simulink model "Electrical_System_2018b_obfs"  (R2019b)
settings: Solver=VariableStepAuto  StartTime=0.0  StopTime=5  RelTol=1e-3  AbsTol=1e-3  EnableMultiTasking=on
InitFcn:
  | Steady_State_Initialisation;
StopFcn:
  | %sscexplore(simlog);
  | %Logging
undefined symbols (not defined in the file): abrlhklxvp, aexgmhuedq, afmfmjnutg, afpphrjpnc, ahuxbyvruc, alarvljztt, amxnyqmnuw, aodrlwvqie, aolhmuplyq, aqpmguuqkg, auesgwirzl, aurophlnng, awamelrhru, ayfhvxflxn, azxkacuhqc, babszerikg, bawhdqanwq, bevoqecvei, bltjvqbchx, bmqsuewujl, bsmyqjfgnf, btvjbsmnve, bywgxqeadw, bziaduxaer, bzmcmdqocb, bzsvyvetat, ccsjnrbsih, cdvenygxwh, cedkrnslhx, cjheorclzs, cjrdshrtqx, ckhavyhcza, ckxewznhlz, cmrcgyiplk, conenicnws, cqkejbgjnn, csfnuwymhe, cunupkhwbh, cwzfvzuxxh, dcadmadufn, dcfponivnv, ddtrqjrhjn, dfhoxvkqas, dfrhtcwpne, dfvomcagjv, djijwylxea, dnmeqksrrm, dnzewbdkaa, dsqcykyxav, dtswwlttmm, ecumpidjtv, edegaywrct, ejjjsmnejc, eknqnehjdz, emvdetzouf, esxbqkbahr, etnkkbreiq, eunoiiiirw, ewewcuedir, fatkfxdhtc ... (+386)
libraries: fl_lib x802, ee_lib x362, fl_ps_legacy_lib x160, nesl_utility x85
(part 10 of 26)

== system Electrical_System_2018b_obfs/Redacted_1221/Redacted_7996/Redacted_1/Redacted_4377/Redacted_6082/Redacted_2183 ==
  Redacted_1396 : fl_lib/Electrical/Electrical Elements/Switch  R_closed=wmcpxqyfeh Ohm  G_open=ordboroxst 1/Ohm  Threshold=puyanqdwrl  i_specify=off  i_priority=None  i=bnajmanprt A  i_nominal_specify=off  i_nominal_unit=A  i_nominal_value=rlbcudmlql  v_specify=off  v_priority=None  v=cqbyhwtmeu V  v_nominal_specify=off  v_nominal_unit=V  v_nominal_value=ssehunbzon
      settings: SourceProductName=Simscape
  Redacted_3366 : ee_lib/Passive/Thermal/Thermal Resistor  R=bawhdqanwq K/W  T_specify=off  T_priority=None  T=nptyawlpaq K  T_nominal_specify=off  T_nominal_unit=K  T_nominal_value=finlbxanjw  Q_specify=off  Q_priority=None  Q=alilpavgri W  Q_nominal_specify=off  Q_nominal_unit=W  Q_nominal_value=wneqapuicx
      settings: SourceProductName=Simscape Electrical  SourceProductBaseCode=PS  InternalSimscapePortConfiguration="{\"Bottom\":[],\"Left\":[{\"id\":\"A\",\"label\":\"A\",\"type\":\"foundation.thermal.thermal\"}],\"Right\":[{\"id\":\"B\",\"label\":\"B\",\"type\":\"foundation.thermal.thermal\"}],\"Top\":[]}"
  Redacted_4085 : fl_lib/Electrical/Electrical Elements/Switch  R_closed=jdqhtjuyba Ohm  G_open=nqhnggplew 1/Ohm  Threshold=jecqzekwwf  i_specify=off  i_priority=None  i=parwtazsiw A  i_nominal_specify=off  i_nominal_unit=A  i_nominal_value=cbscxuyyvd  v_specify=off  v_priority=None  v=prtofmgyxi V  v_nominal_specify=off  v_nominal_unit=V  v_nominal_value=ygccoktkvx
      settings: SourceProductName=Simscape
  Redacted_6327 : ee_lib/Semiconductors & Converters/Diode  ModelType=wmwpyziqse  Vf=hsrvymleww V  Ron=pyrhpbxgop Ohm  Goff=ooooykpefi S  prmExp=fgnltfxrhl  I12=dbygefiygg A  V12=yxnireldoj V  IS=umytqsawsi A  ec=rwknegxugi  I1=qflroumpgm A  V1=riphrjudsb V  RS=tsfshgyhqz Ohm  Tmeas=qkexvrxdoi degC  N_series=cbszsjtyip  N_parallel=ybgzghthgk  Rz=gkwnarnzwz Ohm  BV=yqgteuoupv V  C_param=taxfohzknz  CJ=lmergqmyrh pF  CJ0=qfikrlcnko pF  VJ=zrhpkoalsk V  Mgrad=ztoncwtqia  Vvec=lyykpwvhzi V  Cvec=gasstcbauf pF  FC=eeghpxvwex  Q_param=fnbxqtfxwi  iRM=zmetzqvpxi A  iF=tsqxkbkjzp A  didt=celvxerdut A/us  trr_factor=ciexehbuux  trr=pmnqwrbgch ns  Qrr=rvaiuqfkvk s*uA  TT=lwokilfxpw ns  tau=ydjtzutwsj ns  T_param=rezrybflyz  IS_T2=whhobjfmpx A  I1_T2=fbtorsgebe A  V1_T2=lcyuerboic V  Tmeas2=ffdvqttstk degC  EG_param=qyhjbidgce  EG=sjwyndroxb eV  XTI_param=sliofzfaaf  XTI=sksaqpzvmm  dBVdT=zooqrpscpn V/K  Tdevice=docgwdkzmk degC  i_specify=off  i_priority=None  i=rmpavrhrmg A  i_nominal_specify=off  i_nominal_unit=A  i_nominal_value=sblhgjjhtn  v_specify=off  v_priority=None  v=tqvxxaryfu V  v_nominal_specify=off  v_nominal_unit=V  v_nominal_value=zbwqzplush  i_capacitor_specify=off  i_capacitor_priority=None  i_capacitor=ozsqayjyjj A  i_capacitor_nominal_specify=off  i_capacitor_nominal_unit=A  i_capacitor_nominal_value=bwqctegvbe  v_capacitor_specify=off  v_capacitor_priority=None  v_capacitor=msafonbusr V  v_capacitor_nominal_specify=off  v_capacitor_nominal_unit=V  v_capacitor_nominal_value=alqpnbtqbu  power_dissipated_specify=off  power_dissipated_priority=None  power_dissipated=ldpizezrgb W  power_dissipated_nominal_specify=off  power_dissipated_nominal_unit=W  power_dissipated_nominal_value=jdcvhdvcqn  thermal_network_parameterization=khqyflkkbo  Rth=hbtoumkpux K/W  Rth_Foster=owtwhhuqef K/W  thermal_mass_parameterization=tyagarpfgc  thermal_mass=odjqiqbmnv J/K  thermal_mass_Foster=dpqmogzzyw J/K  thermal_time_constant=nrygysvakb s  thermal_time_constant_Foster=pknwccaesz s  thermal_mass_initial_temperatures=ubqttyiytq degC
      settings: SourceProductName=Simscape Electrical  InternalSimscapePortConfiguration="{\"Bottom\":[],\"Left\":[{\"id\":\"p\",\"label\":\"\",\"type\":\"foundation.electrical.electrical\"},{\"id\":\"H\",\"label\":\"H\",\"type\":\"foundation.thermal.thermal\"}],\"Right\":[{\"id\":\"n\",\"label\":\"\",\"type\":\"foundation.electrical.electrical\"}],\"Top\":[]}"
  Redacted_6920 : ee_lib/Semiconductors & Converters/Diode  ModelType=ifkeajuogy  Vf=rvxoqojvbw V  Ron=wlhpwjfqxp Ohm  Goff=bvtpgzsrrx S  prmExp=nlergzwjbu  I12=cxqwsuomth A  V12=vmavhsfifk V  IS=eyymhspphz A  ec=yiafetqxro  I1=hmubrgwopc A  V1=lmsucbmfuc V  RS=ebxfexknak Ohm  Tmeas=pmaoxtpzfm degC  N_series=kbcwisxpjg  N_parallel=aaklmjotsd  Rz=pkzujcjpob Ohm  BV=gdhqaesgrk V  C_param=qtgcbvllfp  CJ=qsggiorgze pF  CJ0=sddrldehqk pF  VJ=ednypbqmsy V  Mgrad=ynapqanrdu  Vvec=zhnqfijbdq V  Cvec=brtmpahjnt pF  FC=znsqocjczl  Q_param=aczsqxqrku  iRM=kkzlynschx A  iF=weflpmxsur A  didt=ifitwlscxo A/us  trr_factor=cwbxopwcbm  trr=ozwjbkszwz ns  Qrr=tosvjxaqxp s*uA  TT=vwmcrpsobc ns  tau=yavnmcqbxl ns  T_param=bfahnjcmju  IS_T2=iahumvdhta A  I1_T2=omfubwbwfi A  V1_T2=adpnfnmwdl V  Tmeas2=vfowspfngr degC  EG_param=qfnvybezbd  EG=pzpugzngnq eV  XTI_param=acwvpdokxd  XTI=tmjvpeiptd  dBVdT=yiwxmdmzvv V/K  Tdevice=mpkhxzqybm degC  i_specify=off  i_priority=None  i=zsqooaqzpu A  i_nominal_specify=off  i_nominal_unit=A  i_nominal_value=trowwbswpb  v_specify=off  v_priority=None  v=buogftaazb V  v_nominal_specify=off  v_nominal_unit=V  v_nominal_value=qjdjlsbbbw  i_capacitor_specify=off  i_capacitor_priority=None  i_capacitor=siqvzgfjbj A  i_capacitor_nominal_specify=off  i_capacitor_nominal_unit=A  i_capacitor_nominal_value=jygxpnflsn  v_capacitor_specify=off  v_capacitor_priority=None  v_capacitor=auwydfvsni V  v_capacitor_nominal_specify=off  v_capacitor_nominal_unit=V  v_capacitor_nominal_value=ouyytgmkij  power_dissipated_specify=off  power_dissipated_priority=None  power_dissipated=hyulojmtmo W  power_dissipated_nominal_specify=off  power_dissipated_nominal_unit=W  power_dissipated_nominal_value=qbvoqhgkhp  thermal_network_parameterization=ppykqmtlhl  Rth=glausydyft K/W  Rth_Foster=fkytfeohhw K/W  thermal_mass_parameterization=oluvrdypml  thermal_mass=fnhzvqgtxn J/K  thermal_mass_Foster=ppzvcmktwx J/K  thermal_time_constant=dhlpwbmywt s  thermal_time_constant_Foster=gidfxyibkk s  thermal_mass_initial_temperatures=korqzmgtir degC
      settings: SourceProductName=Simscape Electrical  InternalSimscapePortConfiguration="{\"Bottom\":[],\"Left\":[{\"id\":\"p\",\"label\":\"\",\"type\":\"foundation.electrical.electrical\"},{\"id\":\"H\",\"label\":\"H\",\"type\":\"foundation.thermal.thermal\"}],\"Right\":[{\"id\":\"n\",\"label\":\"\",\"type\":\"foundation.electrical.electrical\"}],\"Top\":[]}"
  Redacted_8780 : ee_lib/Passive/Thermal/Thermal Resistor  R=lykhbhfuku K/W  T_specify=off  T_priority=None  T=qujobzntab K  T_nominal_specify=off  T_nominal_unit=K  T_nominal_value=fwjjrigoji  Q_specify=off  Q_priority=None  Q=oyodymkfqm W  Q_nominal_specify=off  Q_nominal_unit=W  Q_nominal_value=ecbnragssr
      settings: SourceProductName=Simscape Electrical  SourceProductBaseCode=PS  InternalSimscapePortConfiguration="{\"Bottom\":[],\"Left\":[{\"id\":\"A\",\"label\":\"A\",\"type\":\"foundation.thermal.thermal\"}],\"Right\":[{\"id\":\"B\",\"label\":\"B\",\"type\":\"foundation.thermal.thermal\"}],\"Top\":[]}"
  Redacted_8981 : ee_lib/Passive/Thermal/Thermal Resistor  R=gcimydvvyd K/W  T_specify=off  T_priority=None  T=seiwuzyrmn K  T_nominal_specify=off  T_nominal_unit=K  T_nominal_value=nxsogkjqln  Q_specify=off  Q_priority=None  Q=iroscqsegj W  Q_nominal_specify=off  Q_nominal_unit=W  Q_nominal_value=bqfmelgyip
      settings: SourceProductName=Simscape Electrical  SourceProductBaseCode=PS  InternalSimscapePortConfiguration="{\"Bottom\":[],\"Left\":[{\"id\":\"A\",\"label\":\"A\",\"type\":\"foundation.thermal.thermal\"}],\"Right\":[{\"id\":\"B\",\"label\":\"B\",\"type\":\"foundation.thermal.thermal\"}],\"Top\":[]}"
  Redacted_9228 : PMIOPort  Side=Left
  Redacted_927 : PMIOPort  Port=2  Side=Left
  Redacted_1010 : PMIOPort  Port=3  Side=Right
  Redacted_500 : PMIOPort  Port=4  Side=Right
  Redacted_1718 : PMIOPort  Port=5  Side=Left
  Redacted_7712 : PMIOPort  Port=6  Side=Right
  connections:
  Redacted_6920/LConn2 -- Redacted_3366/LConn1
  Redacted_8981/RConn1 -- Redacted_1718/RConn1
  Redacted_500/RConn1 -- Redacted_1396/RConn2
  Redacted_4085/RConn1 -- Redacted_1396/RConn1 -- Redacted_7712/RConn1
  Redacted_8780/RConn1 -- Redacted_8981/LConn1 -- Redacted_3366/RConn1
  Redacted_9228/RConn1 -- Redacted_6327/RConn1
  Redacted_6327/LConn1 -- Redacted_4085/LConn1
  Redacted_1010/RConn1 -- Redacted_4085/RConn2
  Redacted_6327/LConn2 -- Redacted_8780/LConn1
  Redacted_6920/RConn1 -- Redacted_1396/LConn1
  Redacted_6920/LConn1 -- Redacted_927/RConn1

== system Electrical_System_2018b_obfs/Redacted_1221/Redacted_7996/Redacted_1/Redacted_4377/Redacted_6082/Redacted_2443 ==
  Neutral_Negative : Subsystem  VariantControl=Variant1
  Positive_Neutral : Subsystem  VariantControl=Variant3
  Redacted_6791 : Subsystem  VariantControl=Variant2
  Redacted_2078 : PMIOPort  Side=Left
  Redacted_827 : PMIOPort  Port=2  Side=Left
  Redacted_65 : PMIOPort  Port=3  Side=Left
  Redacted_2555 : PMIOPort  Port=4  Side=Right
  Redacted_7416 : PMIOPort  Port=5  Side=Right

== system Electrical_System_2018b_obfs/Redacted_1221/Redacted_7996/Redacted_1/Redacted_4377/Redacted_6082/Redacted_248 ==
  Neutral_Negative : Subsystem  VariantControl=Variant1
  Positive_Neutral : Subsystem  VariantControl=Variant3
  Redacted_2281 : Subsystem  VariantControl=Variant2
  Redacted_4518 : PMIOPort  Side=Left
  Redacted_7536 : PMIOPort  Port=2  Side=Left
  Redacted_9561 : PMIOPort  Port=3  Side=Left
  Redacted_1518 : PMIOPort  Port=4  Side=Right
  Redacted_7660 : PMIOPort  Port=5  Side=Right

== system Electrical_System_2018b_obfs/Redacted_1221/Redacted_7996/Redacted_1/Redacted_4377/Redacted_6082/Redacted_2710 ==
  Redacted_1835 : ee_lib/Passive/Thermal/Thermal Resistor  R=zuzrchwspe K/W  T_specify=off  T_priority=None  T=eunoiiiirw K  T_nominal_specify=off  T_nominal_unit=K  T_nominal_value=yftlbkraoc  Q_specify=off  Q_priority=None  Q=kaqhtzlkmw W  Q_nominal_specify=off  Q_nominal_unit=W  Q_nominal_value=kxsmqmphud
      settings: SourceProductName=Simscape Electrical  SourceProductBaseCode=PS  InternalSimscapePortConfiguration="{\"Bottom\":[],\"Left\":[{\"id\":\"A\",\"label\":\"A\",\"type\":\"foundation.thermal.thermal\"}],\"Right\":[{\"id\":\"B\",\"label\":\"B\",\"type\":\"foundation.thermal.thermal\"}],\"Top\":[]}"
  Redacted_2325 : ee_lib/Passive/Thermal/Thermal Resistor  R=oohwiocpwa K/W  T_specify=off  T_priority=None  T=aodrlwvqie K  T_nominal_specify=off  T_nominal_unit=K  T_nominal_value=hbqkshwgbe  Q_specify=off  Q_priority=None  Q=zgbdrenlos W  Q_nominal_specify=off  Q_nominal_unit=W  Q_nominal_value=gyllwstqdw
      settings: SourceProductName=Simscape Electrical  SourceProductBaseCode=PS  InternalSimscapePortConfiguration="{\"Bottom\":[],\"Left\":[{\"id\":\"A\",\"label\":\"A\",\"type\":\"foundation.thermal.thermal\"}],\"Right\":[{\"id\":\"B\",\"label\":\"B\",\"type\":\"foundation.thermal.thermal\"}],\"Top\":[]}"
  Redacted_24 : ee_lib/Semiconductors & Converters/Diode  ModelType=divufniqhz  Vf=fuswyfzioa V  Ron=sfkcggclsz Ohm  Goff=rpmhprrivu S  prmExp=rqsfzusaiw  I12=cqrlsxwtvu A  V12=gimzrykmwg V  IS=rbknwvhbll A  ec=ygxdpgkrus  I1=tarfhsbhda A  V1=auwltsmvvt V  RS=troyncdmko Ohm  Tmeas=dpmoufhgnq degC  N_series=mqgkycpjnt  N_parallel=iatvhhkcmg  Rz=fwzkufafef Ohm  BV=zmpddawwjp V  C_param=qikpakizwp  CJ=hljtvaqupa pF  CJ0=oewuaitods pF  VJ=xrrquippxs V  Mgrad=oyxruwepxk  Vvec=iunesjqkcl V  Cvec=vvxzfuxhsc pF  FC=wwyulevwwe  Q_param=sttqtkaprf  iRM=ykusalgnes A  iF=pvzoejfzxx A  didt=adheigkzej A/us  trr_factor=oeawnjlela  trr=nbebmwvdrw ns  Qrr=lgxgfdaswr s*uA  TT=mupppamadl ns  tau=pradyztspj ns  T_param=djosuqmtzl  IS_T2=kouzrlehuq A  I1_T2=ovjcqjjnvt A  V1_T2=fvujieyhhk V  Tmeas2=epvpjdnelz degC  EG_param=qptvtngyyt  EG=ndvbbapzev eV  XTI_param=msvaynwzcp  XTI=cmxevtkdww  dBVdT=pyfqnygnab V/K  Tdevice=rmrhsufjav degC  i_specify=off  i_priority=None  i=wbjfwxwcps A  i_nominal_specify=off  i_nominal_unit=A  i_nominal_value=npkrcglwju  v_specify=off  v_priority=None  v=pdjfweujkd V  v_nominal_specify=off  v_nominal_unit=V  v_nominal_value=ipmoxmdjvx  i_capacitor_specify=off  i_capacitor_priority=None  i_capacitor=tlbvdlttjz A  i_capacitor_nominal_specify=off  i_capacitor_nominal_unit=A  i_capacitor_nominal_value=lexosykyas  v_capacitor_specify=off  v_capacitor_priority=None  v_capacitor=tjzvbhzdbm V  v_capacitor_nominal_specify=off  v_capacitor_nominal_unit=V  v_capacitor_nominal_value=bewlyffcpp  power_dissipated_specify=off  power_dissipated_priority=None  power_dissipated=uuberenndt W  power_dissipated_nominal_specify=off  power_dissipated_nominal_unit=W  power_dissipated_nominal_value=zxdbkerarj  thermal_network_parameterization=jgdhoyqkgb  Rth=zfnbvvzomp K/W  Rth_Foster=efezaqcttv K/W  thermal_mass_parameterization=dmbasvufig  thermal_mass=tokjdiqqfg J/K  thermal_mass_Foster=mahdpsfuip J/K  thermal_time_constant=zmmzrqwbmo s  thermal_time_constant_Foster=bacfszxpmj s  thermal_mass_initial_temperatures=jgpescfmbb degC
      settings: SourceProductName=Simscape Electrical  InternalSimscapePortConfiguration="{\"Bottom\":[],\"Left\":[{\"id\":\"p\",\"label\":\"\",\"type\":\"foundation.electrical.electrical\"},{\"id\":\"H\",\"label\":\"H\",\"type\":\"foundation.thermal.thermal\"}],\"Right\":[{\"id\":\"n\",\"label\":\"\",\"type\":\"foundation.electrical.electrical\"}],\"Top\":[]}"
  Redacted_467 : ee_lib/Semiconductors & Converters/Diode  ModelType=zwlyghrise  Vf=euzwuqecka V  Ron=sqqlvgrmjb Ohm  Goff=bmldewftqw S  prmExp=fjuhevddso  I12=yyjhzztotg A  V12=uojrvplvvj V  IS=cfmsrmnpsn A  ec=bhxifbozbf  I1=qnabjxlwpe A  V1=qvsekpkmcx V  RS=oaatpqtofx Ohm  Tmeas=fxzrhnbzxw degC  N_series=frjvnwrrls  N_parallel=umpwwncuya  Rz=boqmxjzfda Ohm  BV=vwgvvolkfz V  C_param=wwurieaact  CJ=mhbbjauuqe pF  CJ0=fihxqirexw pF  VJ=kwlcvjkmvx V  Mgrad=wmvcjduqzw  Vvec=eostyisdez V  Cvec=zqwmellhog pF  FC=aywdksybze  Q_param=xegpbnqmsp  iRM=thzcufmasx A  iF=jtqklphmoa A  didt=uaygsalief A/us  trr_factor=hauvgridjf  trr=msqoixcjlj ns  Qrr=tucpeotqzo s*uA  TT=fpdueotkxs ns  tau=uwhowgbepa ns  T_param=yukufyyeby  IS_T2=slesqmfvks A  I1_T2=cyohlfwokl A  V1_T2=zciacdqqef V  Tmeas2=odhefydsxa degC  EG_param=yjfkbklesn  EG=jqezgnscdw eV  XTI_param=etnksvgilo  XTI=pgrzlvrznx  dBVdT=thityipxbq V/K  Tdevice=aamobpecky degC  i_specify=off  i_priority=None  i=knehxtpuza A  i_nominal_specify=off  i_nominal_unit=A  i_nominal_value=tsfgfpsoce  v_specify=off  v_priority=None  v=ztgmiqkbgh V  v_nominal_specify=off  v_nominal_unit=V  v_nominal_value=npuzlaeycc  i_capacitor_specify=off  i_capacitor_priority=None  i_capacitor=tevzevklgo A  i_capacitor_nominal_specify=off  i_capacitor_nominal_unit=A  i_capacitor_nominal_value=ptrppgqifa  v_capacitor_specify=off  v_capacitor_priority=None  v_capacitor=mdzmhpiquf V  v_capacitor_nominal_specify=off  v_capacitor_nominal_unit=V  v_capacitor_nominal_value=dwuxzrnnxv  power_dissipated_specify=off  power_dissipated_priority=None  power_dissipated=maylsgmrfw W  power_dissipated_nominal_specify=off  power_dissipated_nominal_unit=W  power_dissipated_nominal_value=gjltmbkcbk  thermal_network_parameterization=ktvcgskyws  Rth=nrirmgsmli K/W  Rth_Foster=jwhpklzmjv K/W  thermal_mass_parameterization=ocwdrvizwl  thermal_mass=rzcsouwcda J/K  thermal_mass_Foster=ibedqwexgm J/K  thermal_time_constant=rszlxecmsr s  thermal_time_constant_Foster=vuiazerwrm s  thermal_mass_initial_temperatures=jaceaqhftk degC
      settings: SourceProductName=Simscape Electrical  InternalSimscapePortConfiguration="{\"Bottom\":[],\"Left\":[{\"id\":\"p\",\"label\":\"\",\"type\":\"foundation.electrical.electrical\"},{\"id\":\"H\",\"label\":\"H\",\"type\":\"foundation.thermal.thermal\"}],\"Right\":[{\"id\":\"n\",\"label\":\"\",\"type\":\"foundation.electrical.electrical\"}],\"Top\":[]}"
  Redacted_5096 : fl_lib/Electrical/Electrical Elements/Switch  R_closed=bhwptyrbvv Ohm  G_open=yibdhtabty 1/Ohm  Threshold=vyhtmbwtyb  i_specify=off  i_priority=None  i=emdqjvxpbx A  i_nominal_specify=off  i_nominal_unit=A  i_nominal_value=amqougtlub  v_specify=off  v_priority=None  v=txxyluqvej V  v_nominal_specify=off  v_nominal_unit=V  v_nominal_value=rdvslnaxld
      settings: SourceProductName=Simscape
  Redacted_8012 : fl_lib/Electrical/Electrical Elements/Switch  R_closed=anuzxeezmu Ohm  G_open=brgjbcwtyq 1/Ohm  Threshold=smlifqbzgv  i_specify=off  i_priority=None  i=ikjmsfyjtt A  i_nominal_specify=off  i_nominal_unit=A  i_nominal_value=jqmpassdoj  v_specify=off  v_priority=None  v=uwwbrmnmns V  v_nominal_specify=off  v_nominal_unit=V  v_nominal_value=gorbelvbmd
      settings: SourceProductName=Simscape
  Redacted_9794 : ee_lib/Passive/Thermal/Thermal Resistor  R=cmrcgyiplk K/W  T_specify=off  T_priority=None  T=fenyjgxqyv K  T_nominal_specify=off  T_nominal_unit=K  T_nominal_value=lgimuztorp  Q_specify=off  Q_priority=None  Q=ufcrfapicn W  Q_nominal_specify=off  Q_nominal_unit=W  Q_nominal_value=gfckcwtrdf
      settings: SourceProductName=Simscape Electrical  SourceProductBaseCode=PS  InternalSimscapePortConfiguration="{\"Bottom\":[],\"Left\":[{\"id\":\"A\",\"label\":\"A\",\"type\":\"foundation.thermal.thermal\"}],\"Right\":[{\"id\":\"B\",\"label\":\"B\",\"type\":\"foundation.thermal.thermal\"}],\"Top\":[]}"
  Redacted_9473 : PMIOPort  Side=Left
  Redacted_5887 : PMIOPort  Port=2  Side=Left
  Redacted_5665 : PMIOPort  Port=3  Side=Right
  Redacted_3172 : PMIOPort  Port=4  Side=Right
  Redacted_6215 : PMIOPort  Port=5  Side=Left
  Redacted_5523 : PMIOPort  Port=6  Side=Right
  connections:
  Redacted_24/LConn2 -- Redacted_1835/LConn1
  Redacted_2325/RConn1 -- Redacted_6215/RConn1
  Redacted_3172/RConn1 -- Redacted_5096/RConn2
  Redacted_8012/RConn1 -- Redacted_5096/RConn1 -- Redacted_5523/RConn1
  Redacted_9794/RConn1 -- Redacted_2325/LConn1 -- Redacted_1835/RConn1
  Redacted_9473/RConn1 -- Redacted_467/RConn1
  Redacted_467/LConn1 -- Redacted_8012/LConn1
  Redacted_5665/RConn1 -- Redacted_8012/RConn2
  Redacted_467/LConn2 -- Redacted_9794/LConn1
  Redacted_24/RConn1 -- Redacted_5096/LConn1
  Redacted_24/LConn1 -- Redacted_5887/RConn1

== system Electrical_System_2018b_obfs/Redacted_1221/Redacted_7996/Redacted_1/Redacted_4377/Redacted_6082/Redacted_2799 ==
  Redacted_14 : fl_lib/Electrical/Electrical Elements/Switch  R_closed=mmaagsrgbc Ohm  G_open=cicknjhhvm 1/Ohm  Threshold=xnzgccqlwj  i_specify=off  i_priority=None  i=hqzepkyeei A  i_nominal_specify=off  i_nominal_unit=A  i_nominal_value=vodnpbetmk  v_specify=off  v_priority=None  v=flyaivdfjk V  v_nominal_specify=off  v_nominal_unit=V  v_nominal_value=przswfymwq
      settings: SourceProductName=Simscape
  Redacted_256 : fl_lib/Electrical/Electrical Elements/Switch  R_closed=ppwmazeqls Ohm  G_open=zeylpmfzmb 1/Ohm  Threshold=xmbikwqmhm  i_specify=off  i_priority=None  i=ajinaowkbj A  i_nominal_specify=off  i_nominal_unit=A  i_nominal_value=uuuzewolju  v_specify=off  v_priority=None  v=otrqqffjwk V  v_nominal_specify=off  v_nominal_unit=V  v_nominal_value=zwxonvfcbj
      settings: SourceProductName=Simscape
  Redacted_3742 : ee_lib/Passive/Thermal/Thermal Resistor  R=xzmplidnqf K/W  T_specify=off  T_priority=None  T=zshsvjmvwr K  T_nominal_specify=off  T_nominal_unit=K  T_nominal_value=dosrqiwvts  Q_specify=off  Q_priority=None  Q=vqlgxiumlf W  Q_nominal_specify=off  Q_nominal_unit=W  Q_nominal_value=mzjjyrayck
      settings: SourceProductName=Simscape Electrical  SourceProductBaseCode=PS  InternalSimscapePortConfiguration="{\"Bottom\":[],\"Left\":[{\"id\":\"A\",\"label\":\"A\",\"type\":\"foundation.thermal.thermal\"}],\"Right\":[{\"id\":\"B\",\"label\":\"B\",\"type\":\"foundation.thermal.thermal\"}],\"Top\":[]}"
  Redacted_4034 : ee_lib/Passive/Thermal/Thermal Resistor  R=xwkozwvuwb K/W  T_specify=off  T_priority=None  T=hxycofyxfo K  T_nominal_specify=off  T_nominal_unit=K  T_nominal_value=yypnighnae  Q_specify=off  Q_priority=None  Q=mmafkkrzqa W  Q_nominal_specify=off  Q_nominal_unit=W  Q_nominal_value=whndbctdlx
      settings: SourceProductName=Simscape Electrical  SourceProductBaseCode=PS  InternalSimscapePortConfiguration="{\"Bottom\":[],\"Left\":[{\"id\":\"A\",\"label\":\"A\",\"type\":\"foundation.thermal.thermal\"}],\"Right\":[{\"id\":\"B\",\"label\":\"B\",\"type\":\"foundation.thermal.thermal\"}],\"Top\":[]}"
  Redacted_4173 : ee_lib/Semiconductors & Converters/Diode  ModelType=tulmihwegb  Vf=dqomejmcdo V  Ron=wefygixenj Ohm  Goff=cqmqzxrucq S  prmExp=eiicyzsqpu  I12=ayxwizdrlh A  V12=yndzldaqag V  IS=swswswzyjd A  ec=ortvifamwx  I1=xnvlgvzazo A  V1=cbnxrsibxn V  RS=zfzslnafvj Ohm  Tmeas=srzeczzhrz degC  N_series=cwyeowwnyg  N_parallel=rzzndodaag  Rz=tmlorzgljf Ohm  BV=fcdpsvgqfz V  C_param=oxxhjpqmkx  CJ=xdhdpetjne pF  CJ0=eopnboxorm pF  VJ=osjqldaapg V  Mgrad=sntnlkitgv  Vvec=vvvsqyjwlq V  Cvec=faidvknuuq pF  FC=nuslxbnegp  Q_param=wpcsrdqkcn  iRM=epgeeezymy A  iF=qkvtlopthh A  didt=yhywaaqkgu A/us  trr_factor=qlxokqlwik  trr=cfxrlwsbqd ns  Qrr=kjhgrlkgfn s*uA  TT=bdveackwqn ns  tau=qgwpqgtevn ns  T_param=qqwmufuloj  IS_T2=vwhbwynzbb A  I1_T2=ugrcgywvxl A  V1_T2=ofimnalxnp V  Tmeas2=efpyefnltl degC  EG_param=gkihstmgwh  EG=vfradqqcre eV  XTI_param=azeiyqzslh  XTI=jnhjlssjor  dBVdT=ozrkunrvqi V/K  Tdevice=gcqsygldcg degC  i_specify=off  i_priority=None  i=yclnvvlwuv A  i_nominal_specify=off  i_nominal_unit=A  i_nominal_value=eroqkrkcly  v_specify=off  v_priority=None  v=sctiisahnx V  v_nominal_specify=off  v_nominal_unit=V  v_nominal_value=ussldzyupi  i_capacitor_specify=off  i_capacitor_priority=None  i_capacitor=adyhzwaero A  i_capacitor_nominal_specify=off  i_capacitor_nominal_unit=A  i_capacitor_nominal_value=jlugygwjih  v_capacitor_specify=off  v_capacitor_priority=None  v_capacitor=uxlkbyjunk V  v_capacitor_nominal_specify=off  v_capacitor_nominal_unit=V  v_capacitor_nominal_value=zhqwudjppl  power_dissipated_specify=off  power_dissipated_priority=None  power_dissipated=eibromriex W  power_dissipated_nominal_specify=off  power_dissipated_nominal_unit=W  power_dissipated_nominal_value=juxdnssqlz  thermal_network_parameterization=gnvkpcxwlv  Rth=ihxwbqdmwa K/W  Rth_Foster=beymoszazb K/W  thermal_mass_parameterization=bygkjedpev  thermal_mass=rnhkfesbtn J/K  thermal_mass_Foster=zkazddkcub J/K  thermal_time_constant=iaakoydqnw s  thermal_time_constant_Foster=zdtgarfcaf s  thermal_mass_initial_temperatures=ruibdayvoi degC
      settings: SourceProductName=Simscape Electrical  InternalSimscapePortConfiguration="{\"Bottom\":[],\"Left\":[{\"id\":\"p\",\"label\":\"\",\"type\":\"foundation.electrical.electrical\"},{\"id\":\"H\",\"label\":\"H\",\"type\":\"foundation.thermal.thermal\"}],\"Right\":[{\"id\":\"n\",\"label\":\"\",\"type\":\"foundation.electrical.electrical\"}],\"Top\":[]}"
  Redacted_50 : ee_lib/Semiconductors & Converters/Diode  ModelType=tlslewfaay  Vf=peujyhvzuc V  Ron=iinywwhiso Ohm  Goff=lbfktfkkrr S  prmExp=svcvswqzek  I12=pknawufhfo A  V12=ptfuvbychd V  IS=kjqfnojdfy A  ec=flctrxnrxr  I1=ajwjiqbsyg A  V1=dxtuezywhb V  RS=ulheemthex Ohm  Tmeas=sovotrzsqy degC  N_series=kqfrjgkdxt  N_parallel=dhsfhjofpz  Rz=xnzdbvfipb Ohm  BV=kttennmtew V  C_param=trkauaxxgo  CJ=qjuoxphjll pF  CJ0=opijhorsqm pF  VJ=azylszyafb V  Mgrad=fejdgnaumo  Vvec=djwbizfuud V  Cvec=evrqxahnvx pF  FC=yrjvkpzstx  Q_param=stalshewbg  iRM=wudiijvfdv A  iF=nqxlcedqfp A  didt=lntrihncyz A/us  trr_factor=fttzoyjfdv  trr=smhwpttsrx ns  Qrr=ydzomidzbs s*uA  TT=hjyfmfchst ns  tau=enzaztgnrs ns  T_param=gtoiihraka  IS_T2=wgpmdxanuh A  I1_T2=taohkjiidl A  V1_T2=npstajglku V  Tmeas2=jdqghdjeem degC  EG_param=xydbowopwk  EG=eklyxpehqx eV  XTI_param=rffpudgvve  XTI=tirunttxyy  dBVdT=yhduoargvg V/K  Tdevice=gtbwypmaiu degC  i_specify=off  i_priority=None  i=muiumfxgrk A  i_nominal_specify=off  i_nominal_unit=A  i_nominal_value=rjdhepavsq  v_specify=off  v_priority=None  v=keyakrzcyf V  v_nominal_specify=off  v_nominal_unit=V  v_nominal_value=mwcpixjzyg  i_capacitor_specify=off  i_capacitor_priority=None  i_capacitor=qotnunkrph A  i_capacitor_nominal_specify=off  i_capacitor_nominal_unit=A  i_capacitor_nominal_value=gzchpazxzl  v_capacitor_specify=off  v_capacitor_priority=None  v_capacitor=eabcrxaphd V  v_capacitor_nominal_specify=off  v_capacitor_nominal_unit=V  v_capacitor_nominal_value=nssgdlqfnr  power_dissipated_specify=off  power_dissipated_priority=None  power_dissipated=kfsjsdylea W  power_dissipated_nominal_specify=off  power_dissipated_nominal_unit=W  power_dissipated_nominal_value=wnkkrbgvrf  thermal_network_parameterization=gawhesamhy  Rth=raeaeqquga K/W  Rth_Foster=ekchdoiazc K/W  thermal_mass_parameterization=yketfhwoay  thermal_mass=kizpyrkmou J/K  thermal_mass_Foster=noigqejeeh J/K  thermal_time_constant=klaivuzsnk s  thermal_time_constant_Foster=wylcbbwvso s  thermal_mass_initial_temperatures=meuehfpoun degC
      settings: SourceProductName=Simscape Electrical  InternalSimscapePortConfiguration="{\"Bottom\":[],\"Left\":[{\"id\":\"p\",\"label\":\"\",\"type\":\"foundation.electrical.electrical\"},{\"id\":\"H\",\"label\":\"H\",\"type\":\"foundation.thermal.thermal\"}],\"Right\":[{\"id\":\"n\",\"label\":\"\",\"type\":\"foundation.electrical.electrical\"}],\"Top\":[]}"
  Redacted_5032 : fl_lib/Electrical/Electrical Elements/Switch  R_closed=djyuvtcnkf Ohm  G_open=ejggmgjquq 1/Ohm  Threshold=rlxsobzzrp  i_specify=off  i_priority=None  i=vxccvsshfr A  i_nominal_specify=off  i_nominal_unit=A  i_nominal_value=ztoxdgmkab  v_specify=off  v_priority=None  v=mvnjgiecut V  v_nominal_specify=off  v_nominal_unit=V  v_nominal_value=fpxnpgloww
      settings: SourceProductName=Simscape
  Redacted_6997 : ee_lib/Passive/Thermal/Thermal Resistor  R=azxkacuhqc K/W  T_specify=off  T_priority=None  T=iqpeqfrrvo K  T_nominal_specify=off  T_nominal_unit=K  T_nominal_value=kewkgutqyk  Q_specify=off  Q_priority=None  Q=xgacttlsfx W  Q_nominal_specify=off  Q_nominal_unit=W  Q_nominal_value=yrupjjmulu
      settings: SourceProductName=Simscape Electrical  SourceProductBaseCode=PS  InternalSimscapePortConfiguration="{\"Bottom\":[],\"Left\":[{\"id\":\"A\",\"label\":\"A\",\"type\":\"foundation.thermal.thermal\"}],\"Right\":[{\"id\":\"B\",\"label\":\"B\",\"type\":\"foundation.thermal.thermal\"}],\"Top\":[]}"
  Redacted_7122 : ee_lib/Passive/Thermal/Thermal Resistor  R=gequosakke K/W  T_specify=off  T_priority=None  T=yveprcfpax K  T_nominal_specify=off  T_nominal_unit=K  T_nominal_value=vzsojcelwy  Q_specify=off  Q_priority=None  Q=jkflhtqewf W  Q_nominal_specify=off  Q_nominal_unit=W  Q_nominal_value=faocaagqnm
      settings: SourceProductName=Simscape Electrical  SourceProductBaseCode=PS  InternalSimscapePortConfiguration="{\"Bottom\":[],\"Left\":[{\"id\":\"A\",\"label\":\"A\",\"type\":\"foundation.thermal.thermal\"}],\"Right\":[{\"id\":\"B\",\"label\":\"B\",\"type\":\"foundation.thermal.thermal\"}],\"Top\":[]}"
  Redacted_718 : ee_lib/Semiconductors & Converters/Diode  ModelType=hzwalpwpdj  Vf=crtqorbrdf V  Ron=dtuaqqqqfe Ohm  Goff=ssskqvgjwx S  prmExp=rbylebavah  I12=gbcjlilwdj A  V12=owdgltcsjq V  IS=nrrmnrcxhi A  ec=sjfrliwacd  I1=ovljdrbuka A  V1=yrcvmuinuy V  RS=nwffojunvq Ohm  Tmeas=yszihgrhjc degC  N_series=ztkzvvauwc  N_parallel=yvkmyxeqrq  Rz=kkiditdcii Ohm  BV=eaknkoqwmh V  C_param=foimocfbtl  CJ=eiydzmpinc pF  CJ0=mcraqkkuzs pF  VJ=qixoqbkvst V  Mgrad=hddpjyowgv  Vvec=guheqtzurh V  Cvec=kdhksuhaik pF  FC=zxtvmvrhvb  Q_param=fmikkvhfee  iRM=ezawdmxmlz A  iF=gaopzjixqb A  didt=hjkdhyvheh A/us  trr_factor=zvbgvgmece  trr=ztladfgbbr ns  Qrr=ohghveggkt s*uA  TT=lfuileimpg ns  tau=toqwscqzcc ns  T_param=svdrsfxyhd  IS_T2=fcoybgbwvg A  I1_T2=aovrifrckl A  V1_T2=troutbqqfh V  Tmeas2=dvigyfmojm degC  EG_param=cxgsnvltrw  EG=roaclctwok eV  XTI_param=ytrguanjdf  XTI=oldetdbykz  dBVdT=ldyqodwnbm V/K  Tdevice=icnmseucpq degC  i_specify=off  i_priority=None  i=krxbgvsmwo A  i_nominal_specify=off  i_nominal_unit=A  i_nominal_value=gdoveeisns  v_specify=off  v_priority=None  v=blpovjuhzh V  v_nominal_specify=off  v_nominal_unit=V  v_nominal_value=qhvsoswlfe  i_capacitor_specify=off  i_capacitor_priority=None  i_capacitor=sfqremdvkr A  i_capacitor_nominal_specify=off  i_capacitor_nominal_unit=A  i_capacitor_nominal_value=rbthjluwwx  v_capacitor_specify=off  v_capacitor_priority=None  v_capacitor=gvebduyxks V  v_capacitor_nominal_specify=off  v_capacitor_nominal_unit=V  v_capacitor_nominal_value=fjsbamdorq  power_dissipated_specify=off  power_dissipated_priority=None  power_dissipated=ktvjbeqvqd W  power_dissipated_nominal_specify=off  power_dissipated_nominal_unit=W  power_dissipated_nominal_value=cyunqnofah  thermal_network_parameterization=lzdjpskjxw  Rth=tumeaafnqm K/W  Rth_Foster=kqaslzygnv K/W  thermal_mass_parameterization=jflyujjaso  thermal_mass=fpaibrkbgh J/K  thermal_mass_Foster=aldyeqrjbc J/K  thermal_time_constant=criblmxzbw s  thermal_time_constant_Foster=xulbsaulbf s  thermal_mass_initial_temperatures=glkvlbqhly degC
      settings: SourceProductName=Simscape Electrical  InternalSimscapePortConfiguration="{\"Bottom\":[],\"Left\":[{\"id\":\"p\",\"label\":\"\",\"type\":\"foundation.electrical.electrical\"},{\"id\":\"H\",\"label\":\"H\",\"type\":\"foundation.thermal.thermal\"}],\"Right\":[{\"id\":\"n\",\"label\":\"\",\"type\":\"foundation.electrical.electrical\"}],\"Top\":[]}"
  Redacted_763 : ee_lib/Semiconductors & Converters/Diode  ModelType=hdctycuzkw  Vf=tjvifnxfuv V  Ron=cnydbqsicp Ohm  Goff=ducaetsmtv S  prmExp=qgbhzhbvzj  I12=pirpzvgjxh A  V12=dkeprjwegx V  IS=elthpplyto A  ec=bvpbkohuyv  I1=oqczivjaob A  V1=pewfscyzrv V  RS=zgtelmnpgz Ohm  Tmeas=gkesqynpca degC  N_series=ihjpnnbzyc  N_parallel=lsvielbegb  Rz=ysgpebshgc Ohm  BV=atzidqevfp V  C_param=vplbhtrmxb  CJ=dvdyqfgpqq pF  CJ0=hftyrpqher pF  VJ=zurufrrrwz V  Mgrad=hvkdrxkshh  Vvec=kxomedtgot V  Cvec=xexhjpbttn pF  FC=gjtifhglrj  Q_param=mwolqugnqg  iRM=pdvcemnafx A  iF=bxrrdaeako A  didt=jneszdjouz A/us  trr_factor=bcagsmvxms  trr=ajbtpbmsxe ns  Qrr=txpyoxjdma s*uA  TT=fsnskeowqu ns  tau=cvinejynxs ns  T_param=mouvaixcwb  IS_T2=fijgahlnnp A  I1_T2=dybchooyle A  V1_T2=dfdjvdimdv V  Tmeas2=cmxztdcxjs degC  EG_param=ticuubgjcs  EG=jgngctnbnn eV  XTI_param=uttsmqjhgd  XTI=atjgiyfovh  dBVdT=inqkiimwec V/K  Tdevice=fnsyksgizi degC  i_specify=off  i_priority=None  i=gmoioopqlw A  i_nominal_specify=off  i_nominal_unit=A  i_nominal_value=xchzsubtdb  v_specify=off  v_priority=None  v=mjkywipror V  v_nominal_specify=off  v_nominal_unit=V  v_nominal_value=fkgekcnpiq  i_capacitor_specify=off  i_capacitor_priority=None  i_capacitor=icabnwcske A  i_capacitor_nominal_specify=off  i_capacitor_nominal_unit=A  i_capacitor_nominal_value=aehltcuqgt  v_capacitor_specify=off  v_capacitor_priority=None  v_capacitor=vipeafkiog V  v_capacitor_nominal_specify=off  v_capacitor_nominal_unit=V  v_capacitor_nominal_value=qnnlzbcipg  power_dissipated_specify=off  power_dissipated_priority=None  power_dissipated=hvjtajjhyi W  power_dissipated_nominal_specify=off  power_dissipated_nominal_unit=W  power_dissipated_nominal_value=nnxgpbwzip  thermal_network_parameterization=cwisxqftsu  Rth=jjddvozwen K/W  Rth_Foster=aghwyaukad K/W  thermal_mass_parameterization=atgudzouir  thermal_mass=vyptloybls J/K  thermal_mass_Foster=orlfbhuaos J/K  thermal_time_constant=crvhtflimy s  thermal_time_constant_Foster=hlgkgupwbd s  thermal_mass_initial_temperatures=frbaaqknpb degC
      settings: SourceProductName=Simscape Electrical  InternalSimscapePortConfiguration="{\"Bottom\":[],\"Left\":[{\"id\":\"p\",\"label\":\"\",\"type\":\"foundation.electrical.electrical\"},{\"id\":\"H\",\"label\":\"H\",\"type\":\"foundation.thermal.thermal\"}],\"Right\":[{\"id\":\"n\",\"label\":\"\",\"type\":\"foundation.electrical.electrical\"}],\"Top\":[]}"
  Redacted_7641 : ee_lib/Semiconductors & Converters/Diode  ModelType=jvmhhockpn  Vf=lzenknmagk V  Ron=amnubdtfvp Ohm  Goff=qakyhwvous S  prmExp=blzattelof  I12=wpanytdecq A  V12=prkwojorfo V  IS=hgjjhzphes A  ec=oewpcqfnkh  I1=vyspsvooxy A  V1=huknxinpvz V  RS=ywhdnctyml Ohm  Tmeas=blplfcoefb degC  N_series=nklolauvfh  N_parallel=ddnyewkblt  Rz=tyiiogmtyz Ohm  BV=agspwlrier V  C_param=mkgmwbzzdz  CJ=drkywxmhpg pF  CJ0=uxzofloada pF  VJ=festuymhqu V  Mgrad=zdmbswzvpp  Vvec=frqpmlhowi V  Cvec=bzftbnihgf pF  FC=nzktvefmus  Q_param=hzlsxtwhka  iRM=tobfsatnwi A  iF=xgehkjzqvu A  didt=wlzrjxtwwo A/us  trr_factor=qmfgsvlxak  trr=uaffhfasez ns  Qrr=vzqlkowmcn s*uA  TT=dtjsuxjcam ns  tau=vqppzywabh ns  T_param=vmteiodvsc  IS_T2=lyxufzuynr A  I1_T2=lbnpebfcgp A  V1_T2=fzfwfrtqhw V  Tmeas2=vcvnwnitjc degC  EG_param=knnbrzbogx  EG=ongjowqasa eV  XTI_param=ukkzrdnnfh  XTI=rtfbrnjfdp  dBVdT=iiiicbmevw V/K  Tdevice=vugruvdnuy degC  i_specify=off  i_priority=None  i=fiocoldtrl A  i_nominal_specify=off  i_nominal_unit=A  i_nominal_value=vdqgzaympr  v_specify=off  v_priority=None  v=wdejrblydg V  v_nominal_specify=off  v_nominal_unit=V  v_nominal_value=tjexfmbrlj  i_capacitor_specify=off  i_capacitor_priority=None  i_capacitor=xlhegmfnlx A  i_capacitor_nominal_specify=off  i_capacitor_nominal_unit=A  i_capacitor_nominal_value=ddhsbhtaaq  v_capacitor_specify=off  v_capacitor_priority=None  v_capacitor=kguleljzqu V  v_capacitor_nominal_specify=off  v_capacitor_nominal_unit=V  v_capacitor_nominal_value=hfthuvzvxo  power_dissipated_specify=off  power_dissipated_priority=None  power_dissipated=hkwkwlmhpj W  power_dissipated_nominal_specify=off  power_dissipated_nominal_unit=W  power_dissipated_nominal_value=orzrmogzgu  thermal_network_parameterization=ovmhndhqct  Rth=ugrkzxpapn K/W  Rth_Foster=ifwzncieyl K/W  thermal_mass_parameterization=laqtytevyp  thermal_mass=zstpknpqqu J/K  thermal_mass_Foster=yuwesjolvn J/K  thermal_time_constant=iubkltnutk s  thermal_time_constant_Foster=gunwrsxdaj s  thermal_mass_initial_temperatures=rdamugqhty degC
      settings: SourceProductName=Simscape Electrical  InternalSimscapePortConfiguration="{\"Bottom\":[],\"Left\":[{\"id\":\"p\",\"label\":\"\",\"type\":\"foundation.electrical.electrical\"},{\"id\":\"H\",\"label\":\"H\",\"type\":\"foundation.thermal.thermal\"}],\"Right\":[{\"id\":\"n\",\"label\":\"\",\"type\":\"foundation.electrical.electrical\"}],\"Top\":[]}"
  Redacted_8838 : ee_lib/Semiconductors & Converters/Diode  ModelType=cmiwftsvec  Vf=vweaeltcps V  Ron=beemewlmho Ohm  Goff=vavlbwhuvj S  prmExp=azknduoumm  I12=nyugqmmbju A  V12=bmiutjqrlm V  IS=bbpownbwtp A  ec=miqmnxjpgq  I1=sxilebsjza A  V1=esprzkqyxr V  RS=tsmillrglu Ohm  Tmeas=giaemdiozw degC  N_series=ryjyzypeuk  N_parallel=vjdnoyxwil  Rz=nxsivwbwly Ohm  BV=jycrnatugz V  C_param=czpybwxoiu  CJ=jncmqgmwwy pF  CJ0=pszifhxfry pF  VJ=muzqxdetft V  Mgrad=jontdzllgi  Vvec=fyabbwyzfg V  Cvec=hkmxdooefi pF  FC=tjdvovdkcd  Q_param=ebwmwlpwww  iRM=nggbgyzjmm A  iF=esjqdcmydr A  didt=vrwzhcrbri A/us  trr_factor=unnpuhacio  trr=rdcmaojzep ns  Qrr=icmuvztiqq s*uA  TT=xzopqsayzy ns  tau=ksscfjmwbz ns  T_param=gczfiuinnw  IS_T2=jfebpqkhnv A  I1_T2=pammjyvwmu A  V1_T2=stdljyyivk V  Tmeas2=cjmrinkojf degC  EG_param=hoqsreszcq  EG=dsrysbmqlv eV  XTI_param=iijwkinkoy  XTI=hmmsrmdojm  dBVdT=bokdbiybpf V/K  Tdevice=dacdhyyaur degC  i_specify=off  i_priority=None  i=zcbvhyriln A  i_nominal_specify=off  i_nominal_unit=A  i_nominal_value=nraaehjrvw  v_specify=off  v_priority=None  v=lcfhjijqqz V  v_nominal_specify=off  v_nominal_unit=V  v_nominal_value=xvhlohnlhz  i_capacitor_specify=off  i_capacitor_priority=None  i_capacitor=zdqctsrrvi A  i_capacitor_nominal_specify=off  i_capacitor_nominal_unit=A  i_capacitor_nominal_value=ttiqqaiibg  v_capacitor_specify=off  v_capacitor_priority=None  v_capacitor=cauazmmjzr V  v_capacitor_nominal_specify=off  v_capacitor_nominal_unit=V  v_capacitor_nominal_value=phzfwhszym  power_dissipated_specify=off  power_dissipated_priority=None  power_dissipated=qurnfxlckn W  power_dissipated_nominal_specify=off  power_dissipated_nominal_unit=W  power_dissipated_nominal_value=ymbbryiklh  thermal_network_parameterization=mmisqbvuit  Rth=glluhycnqd K/W  Rth_Foster=fkkegkuhwv K/W  thermal_mass_parameterization=tcwdmnlntr  thermal_mass=gpzqevvoni J/K  thermal_mass_Foster=opjuznapoq J/K  thermal_time_constant=hmjjgsgsya s  thermal_time_constant_Foster=rghvfyuwvo s  thermal_mass_initial_temperatures=gqkpqornjx degC
      settings: SourceProductName=Simscape Electrical  InternalSimscapePortConfiguration="{\"Bottom\":[],\"Left\":[{\"id\":\"p\",\"label\":\"\",\"type\":\"foundation.electrical.electrical\"},{\"id\":\"H\",\"label\":\"H\",\"type\":\"foundation.thermal.thermal\"}],\"Right\":[{\"id\":\"n\",\"label\":\"\",\"type\":\"foundation.electrical.electrical\"}],\"Top\":[]}"
  Redacted_5480 : PMIOPort  Side=Left
  Redacted_5609 : PMIOPort  Port=2  Side=Left
  Redacted_8475 : PMIOPort  Port=3  Side=Left
  Redacted_2850 : PMIOPort  Port=4  Side=Right
  Redacted_1993 : PMIOPort  Port=5  Side=Right
  Redacted_7871 : PMIOPort  Port=6  Side=Right
  Redacted_7603 : PMIOPort  Port=7  Side=Left
  Redacted_3441 : PMIOPort  Port=8  Side=Right
  connections:
  Redacted_8838/LConn1 -- Redacted_5609/RConn1 -- Redacted_718/RConn1
  Redacted_8838/RConn1 -- Redacted_256/LConn1 -- Redacted_718/LConn1
  Redacted_3742/LConn1 -- Redacted_763/LConn2 -- Redacted_50/LConn2
  Redacted_2850/RConn1 -- Redacted_5032/RConn2
  Redacted_50/LConn1 -- Redacted_5032/LConn1 -- Redacted_763/RConn1
  Redacted_763/LConn1 -- Redacted_5480/RConn1 -- Redacted_50/RConn1
  Redacted_7122/RConn1 -- Redacted_4034/RConn1 -- Redacted_6997/LConn1 -- Redacted_3742/RConn1
  Redacted_7641/LConn1 -- Redacted_8475/RConn1 -- Redacted_4173/RConn1
  Redacted_7871/RConn1 -- Redacted_14/RConn2
  Redacted_3441/RConn1 -- Redacted_14/RConn1 -- Redacted_256/RConn1 -- Redacted_5032/RConn1
  Redacted_1993/RConn1 -- Redacted_256/RConn2
  Redacted_4173/LConn1 -- Redacted_14/LConn1 -- Redacted_7641/RConn1
  Redacted_4173/LConn2 -- Redacted_4034/LConn1 -- Redacted_7641/LConn2
  Redacted_6997/RConn1 -- Redacted_7603/RConn1
  Redacted_8838/LConn2 -- Redacted_718/LConn2 -- Redacted_7122/LConn1

== system Electrical_System_2018b_obfs/Redacted_1221/Redacted_7996/Redacted_1/Redacted_4377/Redacted_6082/Redacted_2927 ==
  Neutral_Negative : Subsystem  VariantControl=Variant1
  Positive_Neutral : Subsystem  VariantControl=Variant3
  Redacted_9228 : Subsystem  VariantControl=Variant2
  Redacted_7425 : PMIOPort  Side=Left
  Redacted_110 : PMIOPort  Port=2  Side=Left
  Redacted_9932 : PMIOPort  Port=3  Side=Left
  Redacted_5448 : PMIOPort  Port=4  Side=Right
  Redacted_18 : PMIOPort  Port=5  Side=Right

== system Electrical_System_2018b_obfs/Redacted_1221/Redacted_7996/Redacted_1/Redacted_4377/Redacted_6082/Redacted_3086 ==
  Neutral_Negative : Subsystem  VariantControl=Variant1
  Positive_Neutral : Subsystem  VariantControl=Variant3
  Redacted_7741 : Subsystem  VariantControl=Variant2
  Redacted_6054 : PMIOPort  Side=Left
  Redacted_5626 : PMIOPort  Port=2  Side=Left
  Redacted_6271 : PMIOPort  Port=3  Side=Left
  Redacted_2564 : PMIOPort  Port=4  Side=Right
  Redacted_7933 : PMIOPort  Port=5  Side=Right

== system Electrical_System_2018b_obfs/Redacted_1221/Redacted_7996/Redacted_1/Redacted_4377/Redacted_6082/Redacted_3181 ==
  Redacted_1351 : ee_lib/Semiconductors & Converters/Diode  ModelType=seeuamuunc  Vf=tjetfrvgds V  Ron=tkwkxekvdq Ohm  Goff=xzxgjjbiog S  prmExp=tjyqkmyyzz  I12=vfldstogen A  V12=aavwtmhros V  IS=bjqywamhpj A  ec=kdkykdyevk  I1=zmbpaboecy A  V1=udzpdlacpc V  RS=jxlihmcwve Ohm  Tmeas=yyfgspfgbd degC  N_series=zsfxqjbunr  N_parallel=fgwiengsno  Rz=avicgvmlgk Ohm  BV=okerteawrl V  C_param=wbkqkuwogq  CJ=wjeiksybxp pF  CJ0=bhyyzfyxjp pF  VJ=baqqiwdxpe V  Mgrad=ijgrywoabh  Vvec=hkmchzqwjs V  Cvec=boveevrcen pF  FC=zabwgjpoen  Q_param=eawnjzzyvy  iRM=kamsrqwhqk A  iF=gaslkmmfnx A  didt=ntyglgoooi A/us  trr_factor=sysuzqibag  trr=yinnobosjz ns  Qrr=jaajtcswbs s*uA  TT=nsneizmgzk ns  tau=gvehbplkpv ns  T_param=rmggrjeyry  IS_T2=bosnjnhbqx A  I1_T2=sevxlylkmu A  V1_T2=kuctfzdxpm V  Tmeas2=xsehdofiyo degC  EG_param=oeofywqxdk  EG=uifethuxrb eV  XTI_param=wtzpwykpco  XTI=jqlhgbjlia  dBVdT=bvciagvedp V/K  Tdevice=wqvmrlhfms degC  i_specify=off  i_priority=None  i=iibbfecdkw A  i_nominal_specify=off  i_nominal_unit=A  i_nominal_value=rqcvvpbxgl  v_specify=off  v_priority=None  v=ozhvdnmemj V  v_nominal_specify=off  v_nominal_unit=V  v_nominal_value=rgrbkwjmip  i_capacitor_specify=off  i_capacitor_priority=None  i_capacitor=hbcekzmgcv A  i_capacitor_nominal_specify=off  i_capacitor_nominal_unit=A  i_capacitor_nominal_value=hspgnyvvck  v_capacitor_specify=off  v_capacitor_priority=None  v_capacitor=ekhmskymom V  v_capacitor_nominal_specify=off  v_capacitor_nominal_unit=V  v_capacitor_nominal_value=kxjlgmioqp  power_dissipated_specify=off  power_dissipated_priority=None  power_dissipated=edojgqvblt W  power_dissipated_nominal_specify=off  power_dissipated_nominal_unit=W  power_dissipated_nominal_value=tsdphnszae  thermal_network_parameterization=asyzzvkyhi  Rth=lywppooubx K/W  Rth_Foster=vecederauj K/W  thermal_mass_parameterization=fsmsxwodxt  thermal_mass=udhbpbteyl J/K  thermal_mass_Foster=kcaieczpfc J/K  thermal_time_constant=qqooakurgg s  thermal_time_constant_Foster=zxqadwzazc s  thermal_mass_initial_temperatures=ljlpeezqox degC
      settings: SourceProductName=Simscape Electrical  InternalSimscapePortConfiguration="{\"Bottom\":[],\"Left\":[{\"id\":\"p\",\"label\":\"\",\"type\":\"foundation.electrical.electrical\"},{\"id\":\"H\",\"label\":\"H\",\"type\":\"foundation.thermal.thermal\"}],\"Right\":[{\"id\":\"n\",\"label\":\"\",\"type\":\"foundation.electrical.electrical\"}],\"Top\":[]}"
  Redacted_3158 : fl_lib/Electrical/Electrical Elements/Switch  R_closed=hwmyltiiqs Ohm  G_open=oageffilii 1/Ohm  Threshold=llxzcykggr  i_specify=off  i_priority=None  i=towpqqbrgr A  i_nominal_specify=off  i_nominal_unit=A  i_nominal_value=yhnwwkhofb  v_specify=off  v_priority=None  v=qsxecyuspm V  v_nominal_specify=off  v_nominal_unit=V  v_nominal_value=iycquvnywo
      settings: SourceProductName=Simscape
  Redacted_3931 : ee_lib/Semiconductors & Converters/Diode  ModelType=tqxwxbyope  Vf=msvpzzkeba V  Ron=fwkchzqblf Ohm  Goff=svlnqffeyd S  prmExp=mlctstspcp  I12=bbyevmnspz A  V12=uvkidbyuvs V  IS=lpydrxcezd A  ec=qsufrycozn  I1=lepjzvxqxl A  V1=ipknupmupx V  RS=bzinarmuqq Ohm  Tmeas=rkwjjzfkwq degC  N_series=imzifmjoup  N_parallel=wbyltkjjsq  Rz=bisuniwcvj Ohm  BV=jgybmonlsf V  C_param=hbgjuibrwj  CJ=gqvyumecto pF  CJ0=ibsphiesxm pF  VJ=bijqmoevpa V  Mgrad=mubmyiximf  Vvec=byiivkqhni V  Cvec=aoibtvakqs pF  FC=copuhvmvyb  Q_param=bflbuobaow  iRM=zldaqxybvj A  iF=ytnymxtjly A  didt=idoehkwwtj A/us  trr_factor=ebltoywncm  trr=fygpxetjfj ns  Qrr=uimcleybda s*uA  TT=krndejyjuq ns  tau=hukxqqjqto ns  T_param=elgqdsktyc  IS_T2=zbjbtcnzao A  I1_T2=hipcbswwjs A  V1_T2=dsoyluttfa V  Tmeas2=fbupxbajck degC  EG_param=mvsexujbus  EG=xiyujyeecx eV  XTI_param=krdlbkxuyu  XTI=xewpkszqxo  dBVdT=ibvfxirjgx V/K  Tdevice=rknouiddqv degC  i_specify=off  i_priority=None  i=ecenxenwrc A  i_nominal_specify=off  i_nominal_unit=A  i_nominal_value=fxilzhobes  v_specify=off  v_priority=None  v=hrmiwxfjsj V  v_nominal_specify=off  v_nominal_unit=V  v_nominal_value=emarxszixz  i_capacitor_specify=off  i_capacitor_priority=None  i_capacitor=febrtrnqtb A  i_capacitor_nominal_specify=off  i_capacitor_nominal_unit=A  i_capacitor_nominal_value=jccfenurhb  v_capacitor_specify=off  v_capacitor_priority=None  v_capacitor=umlvqkknjw V  v_capacitor_nominal_specify=off  v_capacitor_nominal_unit=V  v_capacitor_nominal_value=gghvoucqhq  power_dissipated_specify=off  power_dissipated_priority=None  power_dissipated=amzqicgaia W  power_dissipated_nominal_specify=off  power_dissipated_nominal_unit=W  power_dissipated_nominal_value=oymruehjkf  thermal_network_parameterization=jpsxuylylh  Rth=uehbhvrzjt K/W  Rth_Foster=tejtqvzged K/W  thermal_mass_parameterization=btxpxztosi  thermal_mass=gxhkmzniwp J/K  thermal_mass_Foster=vdvluvqrgk J/K  thermal_time_constant=idwezoowwk s  thermal_time_constant_Foster=iskjzblkee s  thermal_mass_initial_temperatures=rnchfspvkh degC
      settings: SourceProductName=Simscape Electrical  InternalSimscapePortConfiguration="{\"Bottom\":[],\"Left\":[{\"id\":\"p\",\"label\":\"\",\"type\":\"foundation.electrical.electrical\"},{\"id\":\"H\",\"label\":\"H\",\"type\":\"foundation.thermal.thermal\"}],\"Right\":[{\"id\":\"n\",\"label\":\"\",\"type\":\"foundation.electrical.electrical\"}],\"Top\":[]}"
  Redacted_4404 : ee_lib/Passive/Thermal/Thermal Resistor  R=xexuroemqo K/W  T_specify=off  T_priority=None  T=xnbryopseg K  T_nominal_specify=off  T_nominal_unit=K  T_nominal_value=kdpocicxnp  Q_specify=off  Q_priority=None  Q=hdqjdfbsma W  Q_nominal_specify=off  Q_nominal_unit=W  Q_nominal_value=udkikzuzos
      settings: SourceProductName=Simscape Electrical  SourceProductBaseCode=PS  InternalSimscapePortConfiguration="{\"Bottom\":[],\"Left\":[{\"id\":\"A\",\"label\":\"A\",\"type\":\"foundation.thermal.thermal\"}],\"Right\":[{\"id\":\"B\",\"label\":\"B\",\"type\":\"foundation.thermal.thermal\"}],\"Top\":[]}"
  Redacted_6446 : ee_lib/Passive/Thermal/Thermal Resistor  R=hwqngtoeuw K/W  T_specify=off  T_priority=None  T=hsoozjtrph K  T_nominal_specify=off  T_nominal_unit=K  T_nominal_value=dxhlmwnjse  Q_specify=off  Q_priority=None  Q=nagsetwglx W  Q_nominal_specify=off  Q_nominal_unit=W  Q_nominal_value=cxhyvgnbrj
      settings: SourceProductName=Simscape Electrical  SourceProductBaseCode=PS  InternalSimscapePortConfiguration="{\"Bottom\":[],\"Left\":[{\"id\":\"A\",\"label\":\"A\",\"type\":\"foundation.thermal.thermal\"}],\"Right\":[{\"id\":\"B\",\"label\":\"B\",\"type\":\"foundation.thermal.thermal\"}],\"Top\":[]}"
  Redacted_9048 : ee_lib/Passive/Thermal/Thermal Resistor  R=zjtbpuzrue K/W  T_specify=off  T_priority=None  T=etnkkbreiq K  T_nominal_specify=off  T_nominal_unit=K  T_nominal_value=kahcrnokjt  Q_specify=off  Q_priority=None  Q=lionqndkkr W  Q_nominal_specify=off  Q_nominal_unit=W  Q_nominal_value=rkfkvndftj
      settings: SourceProductName=Simscape Electrical  SourceProductBaseCode=PS  InternalSimscapePortConfiguration="{\"Bottom\":[],\"Left\":[{\"id\":\"A\",\"label\":\"A\",\"type\":\"foundation.thermal.thermal\"}],\"Right\":[{\"id\":\"B\",\"label\":\"B\",\"type\":\"foundation.thermal.thermal\"}],\"Top\":[]}"
  Redacted_9733 : fl_lib/Electrical/Electrical Elements/Switch  R_closed=ovhcdwdqkf Ohm  G_open=owpytlrcdh 1/Ohm  Threshold=yzytgmynyn  i_specify=off  i_priority=None  i=owtxshledt A  i_nominal_specify=off  i_nominal_unit=A  i_nominal_value=nybtewbswk  v_specify=off  v_priority=None  v=kpnujakptf V  v_nominal_specify=off  v_nominal_unit=V  v_nominal_value=jucrzeyoqp
      settings: SourceProductName=Simscape
  Redacted_2911 : PMIOPort  Side=Left
  Redacted_7251 : PMIOPort  Port=2  Side=Left
  Redacted_7245 : PMIOPort  Port=3  Side=Right
  Redacted_1415 : PMIOPort  Port=4  Side=Right
  Redacted_532 : PMIOPort  Port=5  Side=Left
  Redacted_2658 : PMIOPort  Port=6  Side=Right
  connections:
  Redacted_3931/LConn1 -- Redacted_7251/RConn1
  Redacted_3931/RConn1 -- Redacted_3158/LConn1
  Redacted_1351/LConn2 -- Redacted_6446/LConn1
  Redacted_7245/RConn1 -- Redacted_9733/RConn2
  Redacted_1351/LConn1 -- Redacted_9733/LConn1
  Redacted_2911/RConn1 -- Redacted_1351/RConn1
  Redacted_4404/RConn1 -- Redacted_9048/LConn1 -- Redacted_6446/RConn1
  Redacted_2658/RConn1 -- Redacted_3158/RConn1 -- Redacted_9733/RConn1
  Redacted_1415/RConn1 -- Redacted_3158/RConn2
  Redacted_9048/RConn1 -- Redacted_532/RConn1
  Redacted_3931/LConn2 -- Redacted_4404/LConn1

== system Electrical_System_2018b_obfs/Redacted_1221/Redacted_7996/Redacted_1/Redacted_4377/Redacted_6082/Redacted_3818 ==
  Neutral_Negative : Subsystem  VariantControl=Variant1
  Positive_Neutral : Subsystem  VariantControl=Variant3
  Redacted_7647 : Subsystem  VariantControl=Variant2
  Redacted_558 : PMIOPort  Side=Left
  Redacted_9353 : PMIOPort  Port=2  Side=Left
  Redacted_2763 : PMIOPort  Port=3  Side=Left
  Redacted_5509 : PMIOPort  Port=4  Side=Right
  Redacted_3127 : PMIOPort  Port=5  Side=Right

== system Electrical_System_2018b_obfs/Redacted_1221/Redacted_7996/Redacted_1/Redacted_4377/Redacted_6082/Redacted_4174 ==
  Neutral_Negative : Subsystem  VariantControl=Variant1
  Positive_Neutral : Subsystem  VariantControl=Variant3
  Redacted_8370 : Subsystem  VariantControl=Variant2
  Redacted_9679 : PMIOPort  Side=Left
  Redacted_9878 : PMIOPort  Port=2  Side=Left
  Redacted_224 : PMIOPort  Port=3  Side=Left
  Redacted_5953 : PMIOPort  Port=4  Side=Right
  Redacted_7639 : PMIOPort  Port=5  Side=Right

== system Electrical_System_2018b_obfs/Redacted_1221/Redacted_7996/Redacted_1/Redacted_4377/Redacted_6082/Redacted_4278 ==
  Neutral_Negative : Subsystem  VariantControl=Variant1
  Positive_Neutral : Subsystem  VariantControl=Variant3
  Redacted_1592 : Subsystem  VariantControl=Variant2
  Redacted_1495 : PMIOPort  Side=Left
  Redacted_2064 : PMIOPort  Port=2  Side=Left
  Redacted_9467 : PMIOPort  Port=3  Side=Left
  Redacted_1543 : PMIOPort  Port=4  Side=Right
  Redacted_9491 : PMIOPort  Port=5  Side=Right
